simulink model "aufgabe7_sim"  (R2016b)
settings: Solver=VariableStepAuto  StartTime=0.0  StopTime=14  RelTol=1e-3
values from neighbouring files (symbols this model uses):
  ct_o = eye(3)    [aufgabe6.m]    (also in aufgabe7.m = eye(4))
  d_o = [0 0;0 0 ;0 0]    [aufgabe6.m]    (also in aufgabe7.m = [0 0;0 0 ;0 0; 0 0])
  Gamma_o = [gamma, -k_o']    [aufgabe6.m]    (also in aufgabe7.m)
  Phi_o = phi + k_o'*ct(3,:)    [aufgabe6.m]    (also in aufgabe7.m)
  Ta = 10e-03    (= 0.01)    [aufgabe1.m]    (also in aufgabe2.m; aufgabe4.m; aufgabe5.m; aufgabe6.m)
  u_GSM_r = 5.6    [aufgabe2.m]    (also in aufgabe4.m; aufgabe6.m; aufgabe7.m)
  w_P_r = x_R(4)    [aufgabe2.m]    (also in aufgabe4.m = -(R_GSM*d_vP + R_GSM*d_vGSM - (k_GSM^4 + R_GSM^2*d_vP^2 +   ; aufgabe6.m = -(R_GSM*d_vP + R_GSM*d_vGSM - (k_GSM^4 + R_GSM^2*d_vP^2 +   ; aufgabe7.m = -(R_GSM*d_vP + R_GSM*d_vGSM - (k_GSM^4 + R_GSM^2*d_vP^2 +   )
  x_r = [i_GSM_r; phi_GSMP_r; w_GSM_r; w_P_r]    [aufgabe4.m]    (also in aufgabe6.m; aufgabe7.m)
undefined symbols (not defined in the file): c_GSMP, d_cGSM, d_cP, d_GSMP, d_qP, d_vGSM, d_vP, i_GSM_0, J_GSM, J_P, k_GSM, L_GSM, phi_GSMP_0, R_GSM, w_GSM_0, w_P_0
libraries: simulink x1
settings Model: Creator=M  LastModifiedBy=M

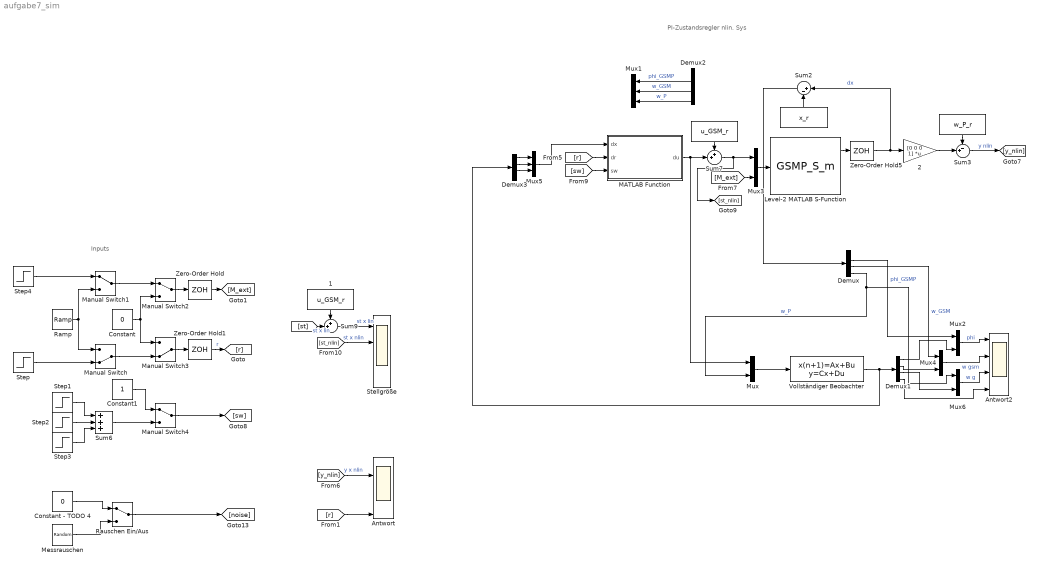
== system aufgabe7_sim ==
  note: Inputs
  note: PI-Zustandsregler nlin. Sys
  " " : Constant  Value=u_GSM_r
  " " : Constant  Value=w_P_r
  " 1" : Constant  Value=u_GSM_r
  " " : Constant  Value=x_r
  "   2" : Gain  Gain=[0 0 0 1]  Multiplication=Matrix(K*u)
  Antwort : Scope  NumInputPorts=5
  Antwort2 : Scope  NumInputPorts=4
  Constant : Constant  Value=0
  Constant - TODO 4 : Constant  Value=0
  Constant1 : Constant
  Demux{,1..3} (4 alike) : Demux
  Level-2 MATLAB S-Function : M-S-Function  FunctionName=GSMP_S_m  Parameters=L_GSM, R_GSM, k_GSM, J_GSM, d_cGSM, d_vGSM, J_P, d_cP, d_vP, d_qP, c_GSMP, d_GSMP, i_GSM_0, phi_GSMP_0, w_GSM_0, w_P_0  mask{L_GSM=L_GSM, R_GSM=R_GSM, k_GSM=k_GSM, J_GSM=J_GSM, d_cGSM=d_cGSM, d_vGSM=d_vGSM, J_P=J_P, d_cP=d_cP, d_vP=d_vP, d_qP=d_qP, c_GSMP=c_GSMP, d_GSMP=d_GSMP, i_GSM_0=i_GSM_0, phi_GSMP_0=phi_GSMP_0, w_GSM_0=w_GSM_0, w_P_0=w_P_0}
      mask prompts: i_GSM_0 "i_GSM"; phi_GSMP_0 "phi_GSMP"; w_GSM_0 "w_GSM"; w_P_0 "w_P"
      mask DialogControl Container3 Prompt: Anfangszustände
  MATLAB Function : MATLAB Function  TreatAsAtomicUnit=on  SystemSampleTime=Ta
  Manual Switch : ManualSwitch  CurrentSetting=0
  Manual Switch1 : ManualSwitch
  Manual Switch2 : ManualSwitch
  Manual Switch3 : ManualSwitch  CurrentSetting=0
  Manual Switch4 : ManualSwitch
  Messrauschen : UniformRandomNumber  Minimum=-5e-2  Maximum=5e-2  SampleTime=1e-3
  Mux{,2..4,6} (5 alike) : Mux  Inputs=2
  Mux1 : Mux  Inputs=3
  Mux5 : Mux  Inputs=3
  Ramp : simulink/Sources/Ramp  slope=1  start=1  X0=0
  Rauschen Ein/Aus : ManualSwitch
  Stellgröße : Scope  NumInputPorts=4
  Step : Step  After=20  SampleTime=0
  Step1 : Step  SampleTime=0
  Step2 : Step  Time=5  After=-1  SampleTime=0
  Step3 : Step  Time=10  SampleTime=0
  Step4 : Step  Time=5  After=-0.5  SampleTime=0
  Sum2 : Sum  Inputs=|+-
  Sum3 : Sum  Inputs=-+|
  Sum6 : Sum  Inputs=+++
  Sum7 : Sum  Inputs=++|
  Sum9 : Sum  Inputs=++|
  Vollständiger Beobachter : DiscreteStateSpace  A=Phi_o  B=Gamma_o  C=ct_o  D=d_o  X0=[0,0,0,0]  SampleTime=Ta
  Zero-Order Hold : ZeroOrderHold  SampleTime=-1
  Zero-Order Hold1 : ZeroOrderHold  SampleTime=-1
  Zero-Order Hold5 : ZeroOrderHold  SampleTime=Ta
  wires:
  Manual Switch1/1 -> Manual Switch2/1
  Constant/1 -> Manual Switch3/1, Manual Switch2/2
  Manual Switch2/1 -> Zero-Order Hold/1
  Manual Switch3/1 -> Zero-Order Hold1/1
  Manual Switch/1 -> Manual Switch3/2
  Ramp/1 -> Manual Switch/1, Manual Switch1/2
  Step/1 -> Manual Switch/2
  Zero-Order Hold1/1 -> [r]  "r"
  Zero-Order Hold/1 -> [M_ext]
  [r] -> Antwort/5
  [r] -> MATLAB Function/2(dr)
  [sw] -> MATLAB Function/3(sw)
  Mux3/1 -> Level-2 MATLAB S-Function/1
  [M_ext] -> Mux3/2
  Zero-Order Hold5/1 -> Sum2/1, "   2"/1  "dx"
  MATLAB Function/1(du) -> Mux/1, Sum7/2
  Sum7/1 -> [st_nlin], Mux3/1
  Demux2/2 -> Mux1/1  "phi_GSMP"
  Demux2/3 -> Mux1/2  "w_GSM"
  Demux2/4 -> Mux1/3  "w_P"
  Sum2/1 -> Demux/1
  Level-2 MATLAB S-Function/1 -> Zero-Order Hold5/1
  "   2"/1 -> Sum3/2
  Sum3/1 -> [y_nlin]  "y nlin"
  Step1/1 -> Sum6/1
  Step2/1 -> Sum6/2
  Step3/1 -> Sum6/3
  Sum6/1 -> Manual Switch4/2
  Manual Switch4/1 -> [sw]
  Constant1/1 -> Manual Switch4/1
  [y_nlin] -> Antwort/2  "y x nlin"
  " "/1 -> Sum7/1
  " "/1 -> Sum3/1
  " "/1 -> Sum2/2
  Messrauschen/1 -> Rauschen Ein/Aus/2
  Constant - TODO 4/1 -> Rauschen Ein/Aus/1
  Rauschen Ein/Aus/1 -> [noise]
  [st_nlin] -> Stellgröße/2  "st x nlin"
  [st] -> Sum9/2  "st x lin"
  " 1"/1 -> Sum9/1
  Sum9/1 -> Stellgröße/1  "st x lin"
  Step4/1 -> Manual Switch1/1
  Demux/2 -> Mux2/1  "phi_GSMP"
  Demux/3 -> Mux4/1  "w_GSM"
  Demux/4 -> Mux6/1, Mux/2  "w_P"
  Mux/1 -> Vollständiger Beobachter/1
  Vollständiger Beobachter/1 -> Demux3/1, Demux1/1
  Mux2/1 -> Antwort2/1  "phi"
  Mux4/1 -> Antwort2/2  "w gsm"
  Mux6/1 -> Antwort2/3  "w g"
  Demux1/1 -> Mux2/2
  Demux1/2 -> Mux4/2
  Demux1/3 -> Mux6/2
  Mux5/1 -> MATLAB Function/1(dx)
  Demux3/1 -> Mux5/1
  Demux3/2 -> Mux5/2
  Demux3/3 -> Mux5/3
  Demux1/4 -> Antwort2/4

== matlab function aufgabe7_sim/MATLAB Function ==
  settings: updateMethod=DISCRETE  sampleTime=0.01
  data: dx input; du output; dr input; sw input; parZR parameter
function du = fcn(dx, dr, sw, parZR)

% Zustand
persistent xI;
if(isempty(xI))
    xI = 0;
end

if (sw~=0)
    yk = parZR.c_z*dx;
    du = [parZR.kx parZR.kI]*[dx; xI] + parZR.kp*(dr - yk);
    
    % xI k+1 berechnen
    xI = xI + (dr - yk);
else
    du = 0;
    xI = 0;
end
